simulink model "DS_distrIntp_4_0_realaxes"  (R2019b)
settings: Solver=FixedStepDiscrete  StartTime=0.0  StopTime=inf  FixedStep=Ts  RelTol=1e-3
StartFcn:
  | close all;
model workspace (MAT data in the model file):
  MvmtPerfEval_collectVal : Simulink.Parameter (value not decoded)
  MvmtPerfEval_sendOwnVal : Simulink.Parameter (value not decoded)
  PAR_center_c2 : Simulink.Parameter (value not decoded)
  PAR_numStepsAheadSmoothing : Simulink.Parameter (value not decoded)
  PAR_startPosReachedTol : Simulink.Parameter (value not decoded)
  PAR_workspace_c2 : Simulink.Parameter (value not decoded)
  PerfEval_numTicks_enable : Simulink.Parameter (value not decoded)
  Segmentregler_I_Gain : Simulink.Parameter (value not decoded)
  Segmentregler_P_Gain : Simulink.Parameter (value not decoded)
  Segmentregler_minVel_enable : Simulink.Parameter (value not decoded)
  Segmentregler_numTicks_enable : Simulink.Parameter (value not decoded)
  Ts : Simulink.Parameter (value not decoded)
  horizon : Simulink.Parameter (value not decoded)
  maxPos_x : Simulink.Parameter (value not decoded)
  maxPos_y : Simulink.Parameter (value not decoded)
  maxPos_z : Simulink.Parameter (value not decoded)
  maxVectorLengths : Simulink.Parameter (value not decoded)
  minAllowedVelSaturation : Simulink.Parameter (value not decoded)
  numAxes : Simulink.Parameter (value not decoded)
  window_length : Simulink.Parameter (value not decoded)
symbols that are objects in the model workspace (value not decoded): MvmtPerfEval_collectVal, MvmtPerfEval_sendOwnVal, numAxes, PAR_center_c2, PAR_numStepsAheadSmoothing, PAR_startPosReachedTol, PAR_workspace_c2, Ts
undefined symbols (not defined in the file or in its folder): DiscIntNeverNeededParam, setP_mat, VelOverride
libraries: vrlib x1, sldrtlib x1
(part 4 of 4)

== stateflow chart DS_distrIntp_4_0_realaxes/Achse X/Chart ==
  state Monitor_Inputs [parallel]
    settings: executionOrder=1
    state Wait
    state Update
      entry:
      send(newCommand);
    (default) -> Monitor_Inputs.Wait
    Monitor_Inputs.Wait -> Update : [hasChanged(ZielPos) ||...
        |  hasChanged(sollGeschw)]
    Update -> Monitor_Inputs.Wait
  state Exec_Commands [parallel]
    settings: executionOrder=2
    state Wait
      during:
      prevZielPos = ZielPos;
    state Send
      entry:
      if prevZielPos > ZielPos && sollGeschw ~= 0
      zP = ZielPos*1000-horizon;
      zP = max(zP,0);
      goToPos(PAR_isAxis,zP,sollGeschw);
      elseif prevZielPos < ZielPos && sollGeschw ~= 0
      zP = ZielPos*1000+horizon;
      goToPos(PAR_isAxis,zP,sollGeschw);
      elseif sollGeschw == 0
      zP = ZielPos *1000;
      goToPos(PAR_isAxis,zP,0.01);
      end
    state Send_after_Start
      % Hier geben wir bei noch icht initialisierter prevZielPos
      % KEINEN Horizont vor, da sonst falscher pos. Offset
      %im ersten Schritt
      entry:
      if prevZielPos > ZielPos && sollGeschw ~= 0
      goToPos(PAR_isAxis,zP,sollGeschw);
      elseif prevZielPos < ZielPos && sollGeschw ~= 0
      goToPos(PAR_isAxis,zP,sollGeschw);
      elseif sollGeschw == 0
      goToPos(PAR_isAxis,zP,0.01);
      end
      startFlag = 0;
    (default) -> Exec_Commands.Wait
    Exec_Commands.Wait -> Send [order 1] : newCommand[startFlag == 0]
    Send -> Exec_Commands.Wait
    Exec_Commands.Wait -> Send_after_Start [order 2] : newCommand
    Send_after_Start -> Exec_Commands.Wait
  state ReadPos [parallel]
    during:
    on every(5,tick): [Pos,TimeStamp] = getPos(PAR_isAxis);
    settings: executionOrder=3
  data: axis function_input; tPos function_input; tVel function_input; pos function_output; axis function_input; timeStamp function_output; ZielPos input; PAR_isAxis input; sollGeschw input; Pos output =0; TimeStamp output =0; prevZielPos local =0; zP local =0; horizon parameter; startFlag local =1
  events: newCommand local FUNCTION_CALL_EVENT
  function goToPos(axis,tPos,tVel):
    | function goToPos(axis,tPos,tVel)
    | 
    | coder.extrinsic('V_2_x_goToPos');
    | V_2_x_goToPos(axis,tPos,tVel);
    | 
    | 
    | end
  function [pos,timeStamp] = getPos(axis):
    | function [pos,timeStamp] = getPos(axis)
    | pos = 0;
    | timeStamp = 0;
    | 
    | coder.extrinsic('V_2_x_getPos');
    | %[pos] = V_2_x_getPos(axis);
    | [pos,timeStamp] = V_2_x_getPos(axis);
    | 
    | end

== stateflow chart DS_distrIntp_4_0_realaxes/Achse Y/Chart ==
  state Monitor_Inputs [parallel]
    settings: executionOrder=1
    state Wait
    state Update
      entry:
      send(newCommand);
    (default) -> Monitor_Inputs.Wait
    Monitor_Inputs.Wait -> Update : [hasChanged(ZielPos) ||...
        |  hasChanged(sollGeschw)]
    Update -> Monitor_Inputs.Wait
  state Exec_Commands [parallel]
    settings: executionOrder=2
    state Wait
      during:
      prevZielPos = ZielPos;
    state Send
      entry:
      if prevZielPos > ZielPos && sollGeschw ~= 0
      zP = ZielPos*1000-horizon;
      zP = max(zP,0);
      goToPos(PAR_isAxis,zP,sollGeschw);
      elseif prevZielPos < ZielPos && sollGeschw ~= 0
      zP = ZielPos*1000+horizon;
      goToPos(PAR_isAxis,zP,sollGeschw);
      elseif sollGeschw == 0
      zP = ZielPos *1000;
      goToPos(PAR_isAxis,zP,0.01);
      end
    state Send_after_Start
      % Hier geben wir bei noch icht initialisierter prevZielPos
      % KEINEN Horizont vor, da sonst falscher pos. Offset
      %im ersten Schritt
      entry:
      if prevZielPos > ZielPos && sollGeschw ~= 0
      goToPos(PAR_isAxis,zP,sollGeschw);
      elseif prevZielPos < ZielPos && sollGeschw ~= 0
      goToPos(PAR_isAxis,zP,sollGeschw);
      elseif sollGeschw == 0
      goToPos(PAR_isAxis,zP,0.01);
      end
      startFlag = 0;
    (default) -> Exec_Commands.Wait
    Exec_Commands.Wait -> Send [order 1] : newCommand[startFlag == 0]
    Send -> Exec_Commands.Wait
    Exec_Commands.Wait -> Send_after_Start [order 2] : newCommand
    Send_after_Start -> Exec_Commands.Wait
  state ReadPos [parallel]
    during:
    on every(5,tick): [Pos,TimeStamp] = getPos(PAR_isAxis);
    settings: executionOrder=3
  data: axis function_input; tPos function_input; tVel function_input; pos function_output; axis function_input; timeStamp function_output; ZielPos input; PAR_isAxis input; sollGeschw input; Pos output =0; TimeStamp output =0; prevZielPos local =0; zP local =0; horizon parameter; startFlag local =1
  events: newCommand local FUNCTION_CALL_EVENT
  function goToPos(axis,tPos,tVel):
    | function goToPos(axis,tPos,tVel)
    | 
    | coder.extrinsic('V_2_x_goToPos');
    | V_2_x_goToPos(axis,tPos,tVel);
    | 
    | 
    | end
  function [pos,timeStamp] = getPos(axis):
    | function [pos,timeStamp] = getPos(axis)
    | pos = 0;
    | timeStamp = 0;
    | 
    | coder.extrinsic('V_2_x_getPos');
    | %[pos] = V_2_x_getPos(axis);
    | [pos,timeStamp] = V_2_x_getPos(axis);
    | 
    | end

== stateflow chart DS_distrIntp_4_0_realaxes/Achse X/Achsgeschwindigkeit ==
  state new_measurement
    entry:
    if(oldTimeStamp) ~= 0
    delta_s = abs(Pos - oldPos);
    delta_t = TimeStamp - oldTimeStamp;
    velocity = delta_s / (delta_t / 1000);
    if sollGeschw ~= 0
    velocity_norm = velocity / (maxVelocity*0.8);
    else
    velocity_norm = 0;
    end
    end
  state Wait_for_new_measurement
    entry:
    oldPos = Pos;
    oldTimeStamp = TimeStamp;
  (default) -> Wait_for_new_measurement
  Wait_for_new_measurement -> new_measurement : [hasChanged(Pos) &&...
      |  hasChanged(TimeStamp)]
  new_measurement -> Wait_for_new_measurement
  data: Pos input; TimeStamp input; velocity output; delta_s local; delta_t local; oldPos local; oldTimeStamp local; velocity_norm output =0; maxVelocity input; sollGeschw input

== stateflow chart DS_distrIntp_4_0_realaxes/Achse Z/Achsgeschwindigkeit ==
  state new_measurement
    entry:
    if(oldTimeStamp) ~= 0
    delta_s = abs(Pos - oldPos);
    delta_t = TimeStamp - oldTimeStamp;
    velocity = delta_s / (delta_t / 1000);
    if sollGeschw ~= 0
    velocity_norm = velocity / (maxVelocity*0.8);
    else
    velocity_norm = 0;
    end
    end
  state Wait_for_new_measurement
    entry:
    oldPos = Pos;
    oldTimeStamp = TimeStamp;
  (default) -> Wait_for_new_measurement
  Wait_for_new_measurement -> new_measurement : [hasChanged(Pos) &&...
      |  hasChanged(TimeStamp)]
  new_measurement -> Wait_for_new_measurement
  data: Pos input; TimeStamp input; velocity output; delta_s local; delta_t local; oldPos local; oldTimeStamp local; velocity_norm output =0; maxVelocity input; sollGeschw input

== stateflow chart DS_distrIntp_4_0_realaxes/Achse Z/Chart ==
  state Monitor_Inputs [parallel]
    settings: executionOrder=1
    state Wait
    state Update
      entry:
      send(newCommand);
    (default) -> Monitor_Inputs.Wait
    Monitor_Inputs.Wait -> Update : [hasChanged(ZielPos) ||...
        |  hasChanged(sollGeschw)]
    Update -> Monitor_Inputs.Wait
  state Exec_Commands [parallel]
    settings: executionOrder=2
    note: Condition ggf. wieder einfügen startFlag == 0
    state Wait
      during:
      prevZielPos = ZielPos;
    state Send
      entry:
      if prevZielPos > ZielPos && sollGeschw ~= 0
      zP = ZielPos*1000-horizon;
      zP = max(zP,0);
      goToPos(PAR_isAxis,zP,sollGeschw);
      elseif prevZielPos < ZielPos && sollGeschw ~= 0
      zP = ZielPos*1000+horizon;
      goToPos(PAR_isAxis,zP,sollGeschw);
      elseif sollGeschw == 0
      zP = ZielPos *1000;
      goToPos(PAR_isAxis,zP,0.01);
      end
    state Send_after_Start [commented out]
      % Hier geben wir bei noch icht initialisierter prevZielPos
      % KEINEN Horizont vor, da sonst falscher pos. Offset
      %im ersten Schritt
      entry:
      if prevZielPos > ZielPos && sollGeschw ~= 0
      goToPos(PAR_isAxis,zP,sollGeschw);
      elseif prevZielPos < ZielPos && sollGeschw ~= 0
      goToPos(PAR_isAxis,zP,sollGeschw);
      elseif sollGeschw == 0
      goToPos(PAR_isAxis,zP,0.01);
      end
      startFlag = 0;
    (default) -> Exec_Commands.Wait
    Exec_Commands.Wait -> Send : newCommand
    Send -> Exec_Commands.Wait
    Exec_Commands.Wait -> Send_after_Start [commented out] : newCommand
    Send_after_Start -> Exec_Commands.Wait [commented out]
  state ReadPos [parallel]
    during:
    on every(5,tick): [Pos,TimeStamp] = getPos(PAR_isAxis);
    settings: executionOrder=3
  data: axis function_input; tPos function_input; tVel function_input; pos function_output; axis function_input; timeStamp function_output; ZielPos input; PAR_isAxis input; sollGeschw input; Pos output =0; TimeStamp output =0; prevZielPos local =0; zP local =0; horizon parameter; startFlag local =1
  events: newCommand local FUNCTION_CALL_EVENT
  function goToPos(axis,tPos,tVel):
    | function goToPos(axis,tPos,tVel)
    | 
    | coder.extrinsic('V_2_x_goToPos');
    | V_2_x_goToPos(axis,tPos,tVel);
    | 
    | 
    | end
  function [pos,timeStamp] = getPos(axis):
    | function [pos,timeStamp] = getPos(axis)
    | pos = 0;
    | timeStamp = 0;
    | 
    | coder.extrinsic('V_2_x_getPos');
    | %[pos] = V_2_x_getPos(axis);
    | [pos,timeStamp] = V_2_x_getPos(axis);
    | 
    | end

== stateflow chart DS_distrIntp_4_0_realaxes/Velocity GUI/Chart ==
  state Default
    during:
    %vel_x = GET_istGeschw(1);
    %vel_y = GET_istGeschw(2);
    %vel_z = GET_istGeschw(3);
    %vel_ges = sqrt(vel_x^2 + vel_y^2 + vel_z^2);
    vel_x_OR = VelOverride(1)*100;
    vel_y_OR = VelOverride(2)*100;
    vel_z_OR = VelOverride(3)*100;
    vel_c2_OR = VelOverride(4)*100;
    vel_ges = vecnorm(GET_normGeschw)*100;
    vel_ges_OR = vecnorm(VelOverride*100);
    vel_x_norm = min(GET_normGeschw(1)*100,vel_x_OR);
    vel_y_norm = min(GET_normGeschw(2)*100,vel_y_OR);
    vel_z_norm = min(GET_normGeschw(3)*100,vel_z_OR);
    vel_c2_norm = min(GET_normGeschw(4)*100,vel_c2_OR);
  (default) -> Default
  data: VelOverride data_store_memory; GET_istGeschw data_store_memory; GET_normGeschw data_store_memory; vel_ges output; vel_ges_OR output; vel_x_norm output; vel_y_norm output; vel_z_norm output; vel_x_OR output; vel_y_OR output; vel_z_OR output; vel_c2_OR output; vel_c2_norm output

== stateflow chart DS_distrIntp_4_0_realaxes/PosTracer ==
  state Wait_for_Init
  state Create_Plot
    entry:
    startPos = PS_createTracePlot(numAxes,PAR_workspace_c2./1000,PAR_center_c2./1000);
  state Fetch_Positions
    entry:
    for ii=1:size(GET_istPos,1)
    switch ii
    case 1
    pos_x = GET_istPos(ii);
    case 2
    pos_y = GET_istPos(ii);
    case 3
    pos_z = GET_istPos(ii);
    case 4
    pos_c2 = GET_istPos(ii);
    c2_RUN = 0 ~= GET_normGeschw(ii);
    case 5
    pos_x2 = GET_istPos(ii);
    end
    end
  state Update_Plot
    entry:
    if numAxes == 2
    PS_updateTracePlot(numAxes,pos_x,pos_y,0,0,0,FLAG_axesRunning,...
    PAR_workspace_c2,PAR_center_c2, c2_RUN);
    elseif numAxes == 3
    PS_updateTracePlot(numAxes,pos_x,pos_y,...
    pos_z,0,0,FLAG_axesRunning,PAR_workspace_c2,PAR_center_c2, c2_RUN);
    elseif numAxes == 4
    PS_updateTracePlot(numAxes,pos_x,pos_y,...
    pos_z,pos_c2,0,FLAG_axesRunning,PAR_workspace_c2,...
    PAR_center_c2, c2_RUN);
    elseif numAxes == 5
    PS_updateTracePlot(numAxes,pos_x,pos_y,...
    pos_z,pos_c2,pos_x2,FLAG_axesRunning,...
    PAR_workspace_c2,PAR_center_c2, c2_RUN);
    end
  state Update_Plot1 [commented out]
    entry:
    if numAxes == 2
    PS_updateTracePlot(numAxes,pos_x+startPos(1,1),pos_y+startPos(1,2),0,0,0,false,...
    PAR_workspace_c2./1000,PAR_center_c2./1000);
    elseif numAxes == 3
    PS_updateTracePlot(numAxes,pos_x+startPos(1,1),pos_y+startPos(1,2),...
    pos_z+startPos(1,3),0,0,true,PAR_workspace_c2./1000,PAR_center_c2./1000);
    elseif numAxes == 4
    PS_updateTracePlot(numAxes,pos_x+startPos(1,1),pos_y+startPos(1,2),...
    pos_z+startPos(1,3),pos_c2+startPos(1,4),0,true,PAR_workspace_c2./1000,...
    PAR_center_c2./1000);
    elseif numAxes == 5
    PS_updateTracePlot(numAxes,pos_x+startPos(1,1),pos_y+startPos(1,2),...
    pos_z+startPos(1,3),pos_c2+startPos(1,4),pos_x2+startPos(1,5),true,...
    PAR_workspace_c2./1000,PAR_center_c2./1000);
    end
  (default) -> Wait_for_Init
  Wait_for_Init -> Create_Plot : after(0.1,'sec')
  Create_Plot -> Fetch_Positions
  Fetch_Positions -> Update_Plot
  Update_Plot -> Fetch_Positions : after(15,tick)
  data: numAx function_input; sPos function_output; c2Workspace function_input; c2Center function_input; numAx function_input; pos1 function_input; pos2 function_input; pos3 function_input; pos4 function_input; pos5 function_input; drawLine function_input; c2Workspace function_input; c2Center function_input; c2_isRunning function_input; numAxes parameter; pos_x local =0; pos_y local =0; GET_istPos data_store_memory; pos_z local =0; startPos local size=[1 numAxes] =zeros(1,numAxes); ii local; bootstrapping_done local; pos_c2 local; pos_x2 local; PAR_center_c2 parameter; PAR_workspace_c2 parameter; GET_normGeschw data_store_memory; c2_RUN local; FLAG_axesRunning data_store_memory
  function sPos  = PS_createTracePlot(numAx,c2Workspace,c2Center):
    | function sPos  = PS_createTracePlot(numAx,c2Workspace,c2Center)
    | 
    | coder.extrinsic('evalin');
    | coder.extrinsic('setappdata');
    | 
    | setP = evalin('base','setP_mat');
    | 
    | sPos = zeros(1,numAx);
    | 
    | % x2Center = [450,75,1]; %x,y,z
    | % x2Workspace = [300,5,2]; %x-wide,y-wide,z-wide
    | 
    | % if(numAx == 5)
    | %     fig = figure;
    | %     ax = axes;
    | %         
    | %     [~,dim2,~] = size(setP);
    | %     plot3(ax,setP(1,1:dim2),setP(2,1:dim2),setP(3,1:dim2));
    | %     hold on
    | %     s = linspace(0,2*pi,50);
    | %     cX = [c2Center(1) (cos(s).*(c2Workspace(4)+c2Workspace(5))/2+c2Center(1))];
    | % 	cY = [c2Center(2) (-sin(s).*(c2Workspace(4)+c2Workspace(5))/2+c2Center(2))];
    | %     cZ = ones(1,length(cX)).*c2Center(3);
    | %     plot3(cX,cY,cZ);
    | %     hold on
    | %     x2X = linspace(x2Center(1)-x2Workspace(1)/2,x2Center(1)+x2Workspace(1)/2);
    | %     x2Y = ones(1,length(x2X)).*x2Center(2);
    | %     x2Z = ones(1,length(x2X)).*x2Center(3);
    | %     plot3(x2X,x2Y,x2Z); 
    | %     hold off
    | %     
    | %     
    | %     set(fig,'Tag','TraceFig');
    | %     set(ax,'Tag','TraceAxes');
    | %     set(ax,'NextPlot','add');
    | %     
    | %     sPos(1,1) = setP(1,1);
    | %     sPos(1,2) = setP(2,1);
    | %     sPos(1,3) = setP(3,1);
    | %     sPos(1,4) = 0;
    | %     sPos(1,5) = x2Center(1)-x2Workspace(1)/2;
    | %     
    | %     traceLine = plot3(ax,[setP(1,1) setP(1,1)],[setP(2,1) setP(2,1)],[setP(3,1) setP(3,1)],'Color',[0 0 1],'LineWidth',1);
    | %     setappdata(ax,'traceLine',traceLine);
    | 
    | if(numAx == 4)
    |     fig = figure;
    |     ax = axes;
    | 
    |         
    |     % Darstellung der Solltrajektorie
    |     [~,dim2,~] = size(setP);
    |     plot3(ax,setP(1,1:dim2),setP(2,1:dim2),setP(3,1:dim2),'k');
    | %     hold on
    |     set(ax,'NextPlot','add');  
    |     
    |     % Darstellung des RT
    |     s = linspace(0,2*pi,50);
    |     radius = (c2Workspace(4)+c2Workspace(5))/2;
    |     cX = [c2Center(1) (cos(s).*radius+c2Center(1))] .* 1000;
    | 	cY = [c2Center(2) (-sin(s).*radius+c2Center(2))] .* 1000;
    |     cZ1 = ones(1,length(cX)).*(c2Center(3)+c2Workspace(3)/2) .* 1000;
    |     plotKreis1 = plot3(ax,cX(2:end),cY(2:end),cZ1(2:end),'g', 'LineWidth', 5); 
    | %     hold off
    | %     cZ2 = ones(1,length(cX)).*(c2Center(3)-c2Workspace(3)/2) .* 1000;
    | %     plotKreis2 = plot3(ax,cX,cY,cZ2);
    |     
    |     set(fig,'Name','Verteilte Interpolation - DEVEKOS');
    |     set(fig, 'Position',  [0, 0, 1450, 1000]) % 1920 x 1080 px sind verfügbar
    |     set(fig,'MenuBar','none');
    |     set(fig,'ToolBar','none');
    |     set(ax, 'ZLim', [-0.01 0.08]) ;
    |     set(fig,'Tag','TraceFig');
    |     set(ax,'Tag','TraceAxes');
    |     set(ax,'ZDir','reverse');
    |     set(ax,'YDir','reverse');
    | 
    | 
    |     
    |     sPos(1,1) = setP(1,1);
    |     sPos(1,2) = setP(2,1);
    |     sPos(1,3) = setP(3,1);
    |     sPos(1,4) = 0;
    |     
    |     traceLine = plot3(ax,[setP(1,1) setP(1,1)],[setP(2,1) setP(2,1)],[setP(3,1) setP(3,1)],'Color',[0 0 1],'LineWidth',1);
    |     setappdata(ax,'traceLine',traceLine);
    | 
    | elseif(numAx == 3)
    |     fig = figure;
    |     ax = axes;
    |         
    |     [~,dim2,~] = size(setP);
    |     plot3(ax,setP(1,1:dim2),setP(2,1:dim2),setP(3,1:dim2));
    |     
    |     set(fig,'Tag','TraceFig');
    |     set(ax,'Tag','TraceAxes');
    |     set(ax,'NextPlot','add');
    |     
    |     sPos(1,1) = setP(1,1);
    |     sPos(1,2) = setP(2,1);
    |     sPos(1,3) = setP(3,1);
    |     
    |     traceLine = plot3(ax,[setP(1,1) setP(1,1)],[setP(2,1) setP(2,1)],[setP(3,1) setP(3,1)],'Color',[0 0 1],'LineWidth',1);
    |     setappdata(ax,'traceLine',traceLine);
    |     
    | elseif(numAx == 2)
    |     
    |     fig = figure;
    |     ax = axes;
    |         
    |     [~,dim2] = size(setP);
    |     plot(ax,setP(1,1:dim2),setP(2,1:dim2));
    |     
    |     set(fig,'Tag','TraceFig');
    |     set(ax,'Tag','TraceAxes');
    |     set(ax,'NextPlot','add');
    |     
    |     sPos(1,1) = setP(1,1);
    |     sPos(1,2) = setP(2,1);
    |     
    |     traceLine = plot(ax,[setP(1,1) setP(1,1)],[setP(2,1) setP(2,1)],'Color',[0 0 1],'LineWidth',1);
    |     setappdata(ax,'traceLine',traceLine);
    |     
    | end
    | 
    | 
    | end
  function PS_updateTracePlot(numAx,pos1,pos2,pos3,pos4,pos5,drawLine,c2Workspace,c2Center, c2_isRunning):
    | function PS_updateTracePlot(numAx,pos1,pos2,pos3,pos4,pos5,drawLine,c2Workspace,c2Center, c2_isRunning)
    | 
    | cRadius = (c2Workspace(4)+c2Workspace(5))/2;
    | markersize=75;
    | % x2Center = [450,75,1]; %x,y,z
    | % x2Workspace = [300,5,2]; %x-wide,y-wide,z-wide
    | 
    | coder.extrinsic('delete');
    | coder.extrinsic('scatter');
    | coder.extrinsic('scatter3');
    | coder.extrinsic('getappdata');
    | coder.extrinsic('setappdata');
    | 
    | ax = findobj('Tag','TraceAxes');
    | 
    | 
    | if(numAx >= 3)
    |     
    |     punkt = getappdata(ax,'tracePunkt');
    |     if isempty(punkt)
    |         punkt = scatter3(ax,pos1,pos2,pos3,markersize,'MarkerEdgeColor','r','LineWidth',2.5);
    |         setappdata(ax,'tracePunkt',punkt);
    |     else
    |         set(punkt,'XData',pos1);
    |         set(punkt,'YData',pos2);
    |         set(punkt,'ZData',pos3);
    |         if c2_isRunning
    |             set(punkt,'MarkerEdgeColor', 'g');
    |         else
    |             set(punkt,'MarkerEdgeColor', 'r');
    |         end
    |             
    |     end
    |     
    |     
    |     colvec=['m','r','g','b','y','k'];
    |     if (numAx >= 4)
    |         for i=1:6
    |             formatSpec = 'tracePunktC%d';
    |             punktC = getappdata(ax,sprintf(formatSpec,cast(i,'int8')));
    |             xKoord = c2Center(1) - cos((pos4+i*60-60)/180*pi)*cRadius;
    |             yKoord = -(c2Center(2) + sin((pos4+i*60-60)/180*pi)*cRadius)+2*c2Center(2);
    |             if isempty(punktC)
    |                 punktC = scatter3(ax,xKoord,yKoord,(c2Center(3)+c2Workspace(3)/2), markersize, 'MarkerEdgeColor','k','LineWidth',2.5);
    |                 setappdata(ax,sprintf(formatSpec,cast(i,'int8')),punktC);
    |             else
    |                 set(punktC,'XData',xKoord);
    |                 set(punktC,'YData',yKoord);
    |             end
    |             % SynchLine zeichnen
    |                 if drawLine && c2_isRunning
    |                     if  i == 5
    |                        synch = getappdata(ax,'synchLine');
    |                         if  isempty(synch)
    |                             synch = plot3(ax, [pos1, xKoord], [pos2, yKoord], [pos3, (c2Center(3)+c2Workspace(3)/2)],':g', 'LineWidth',2.5);
    |                             setappdata(ax,'synchLine',synch);
    |                         else
    |                             set(synch,'XData',[pos1, xKoord]);
    |                             set(synch,'YData',[pos2, yKoord]);
    |                             set(synch,'ZData',[pos3, (c2Center(3)+c2Workspace(3)/2)]);
    |                         end
    |                     end
    |                 else
    |                     synch = getappdata(ax,'synchLine');
    |         
    |                     set(synch,'XData',[]);
    |                     set(synch,'YData',[]);
    |                     set(synch,'ZData',[]);
    |                 end  
    | 
    |             
    |         end
    |         
    | %         if (numAx >= 5)
    | %             punktX2 = getappdata(ax,'tracePunktX2');
    | %             if isempty(punktX2)
    | %                 punktX2 = scatter3(ax,pos5,75,0,'MarkerEdgeColor','g','LineWidth',1.5);
    | %                 setappdata(ax,'tracePunktX2',punktX2);
    | %             else
    | %                 set(punktX2,'XData',pos5);
    | %             end
    | %         end
    |     end
    |     
    |     if drawLine
    |         
    |         traceLine = getappdata(ax,'traceLine');
    |         XData = get(traceLine,'XData');
    |         YData = get(traceLine,'YData');
    |         ZData = get(traceLine,'ZData');
    |         
    |         set(traceLine,'LineWidth',5);
    |         set(traceLine,'XData',[XData pos1]);
    |         set(traceLine,'YData',[YData pos2]);
    |         set(traceLine,'ZData',[ZData pos3]);
    |         
    |     else
    |         
    |         traceLine = getappdata(ax,'traceLine');
    |         
    |         set(traceLine,'XData',[]);
    |         set(traceLine,'YData',[]);
    |         set(traceLine,'ZData',[]);
    |         
    |     end
    |     
    | elseif(numAx == 2)
    |     
    |     punkt = scatter(ax,pos1,pos2,'MarkerEdgeColor','r','LineWidth',2);
    |     setappdata(ax,'tracePunkt',punkt);
    |     
    |     if drawLine
    |         
    |         traceLine = getappdata(ax,'traceLine');
    |         XData = get(traceLine,'XData');
    |         YData = get(traceLine,'YData');
    |         
    |         set(traceLine,'XData',[XData pos1]);
    |         set(traceLine,'YData',[YData pos2]);
    |         
    |     end   
    | end
    | end

== stateflow chart DS_distrIntp_4_0_realaxes/Joystick Ctrl/Chart ==
  state Idle
  state Start_interpolation
    entry:
    FLAG_startButton = true;
  state Stop_interpolation
    entry:
    FLAG_stopButton = true;
  note: Knopf
      | Zuordnung
      |
      | B(1)
      | Knopf A
      |
      | B(2)
      | Knopf B
      |
      | B(3)
      | Knopf X
      |
      | B(4)
      | Knopf Y
      |
      | B(5)
      | Knopf LB
      |
      | B(6)
      | Knopf RB
      |
      | B(7)
      | Knopf Reset
      |
      | B(8)
      | Knopf Start
      |
      | B(9)
      | Druckpunkt linker Stick
  note: Achse
      | Zuordnung
      |
      | A(1)
      | linker Stick (horizontal)
      |
      | A(2)
      | linker Stick (vertikal)
      |
      | A(3)
      | Trigger
      |
      | A(4)
      | rechter Stick (horizontal)
      |
      | A(5)
      | rechter Stick (vertikal)
  state Override_anpassen
    during:
    orX(1) = B(3)*A(3);
    orY(1) = B(4)*A(3);
    orZ(1) = B(1)*A(3);
    orC2(1) = B(2)*A(3);
    exit:
    orX(1) = 0;
    orY(1) = 0;
    orZ(1) = 0;
    orC2(1) = 0;
  state Override_gesamt_Reset
    entry:
    orX(2) = 1;
    orY(2) = 1;
    orZ(2) = 1;
    orC2(2) = 1;
    exit:
    orX(2) = 0;
    orY(2) = 0;
    orZ(2) = 0;
    orC2(2) = 0;
  state Override_Achse_Reset
    state axX
      entry:
      FLAG_resetAxis(1) = 1;
      FLAG_stopButton = true;
    state axY
      entry:
      FLAG_resetAxis(2) = 1;
      FLAG_stopButton = true;
    state axZ
      entry:
      FLAG_resetAxis(3) = 1;
      FLAG_stopButton = true;
    (junction 30) -> axZ [order 3] : [B(1)]
    (junction 30) -> axX [order 1] : [B(3)]
    (junction 30) -> axY [order 2] : [B(4)]
  (default) -> Idle
  Idle -> Start_interpolation [order 4] : [B(8) == 1]
  Start_interpolation -> Idle : [B(8) == 0]
  Idle -> Stop_interpolation [order 5] : [B(7) == 1]
  Stop_interpolation -> Idle : [B(7) == 0]
  Idle -> Override_anpassen [order 3] : [(B(1) || B(3) || B(4)) || B(2) && B(5) ~=1 && B(6)~=1]
  Override_anpassen -> Idle : [B(1)==0 && B(3)==0 && B(4)==0 && B(2) == 0]
  Idle -> Override_gesamt_Reset [order 2] : [B(9)]
  Override_gesamt_Reset -> Idle
  Idle -> (junction 30) [order 1] : [B(5) && B(6)]
  Override_Achse_Reset -> Idle : [B(5) == 0 || B(6) == 0]
  data: A input; orX output size=[1 2] =[0 0]; B input; orY output size=[1 2] =[0 0]; orZ output size=[1,2] =[0 0]; FLAG_startButton data_store_memory; FLAG_stopButton data_store_memory; FLAG_resetAxis data_store_memory; orC2 output size=[1,2] =[0 0]

== stateflow chart DS_distrIntp_4_0_realaxes/Joystick Ctrl/Chart1 ==
  state Idle
    JoystickTT();
  note: Knopf
      | Zuordnung
      |
      | B(1)
      | Knopf A
      |
      | B(2)
      | Knopf B
      |
      | B(3)
      | Knopf X
      |
      | B(4)
      | Knopf Y
      |
      | B(5)
      | Knopf LB
      |
      | B(6)
      | Knopf RB
      |
      | B(7)
      | Knopf Reset
      |
      | B(8)
      | Knopf Start
  note: Achse
      | Zuordnung
      |
      | A(1)
      | linker Stick (horizontal)
      |
      | A(2)
      | linker Stick (vertikal)
      |
      | A(3)
      | Trigger
      |
      | A(4)
      | rechter Stick (horizontal)
      |
      | A(5)
      | rechter Stick (vertikal)
  (default) -> Idle
  data: A input; orX output size=[1 2] =[0 0]; B input; orY output size=[1 2] =[0 0]; orZ output size=[1,2] =[0 0]; FLAG_stopButton data_store_memory; FLAG_startButton data_store_memory
  function JoystickTT:
    | function JoystickTT
    | 
    | aVarTruthTableCondition_1 = false;
    | aVarTruthTableCondition_2 = false;
    | aVarTruthTableCondition_3 = false;
    | aVarTruthTableCondition_4 = false;
    | aVarTruthTableCondition_5 = false;
    | aVarTruthTableCondition_6 = false;
    | aVarTruthTableCondition_7 = false;
    | aVarTruthTableCondition_8 = false;
    | 
    | 
    | % Knopf X
    | % (x-Achse)
    | 
    | aVarTruthTableCondition_1 = logical(B(3));
    | 
    | % Knopf Y
    | % (y-Achse)
    | 
    | aVarTruthTableCondition_2 = logical(B(4));
    | 
    | % Knopf A
    | % (z-Achse)
    | 
    | aVarTruthTableCondition_3 = logical(B(1));
    | 
    | % Knopf B
    | 
    | aVarTruthTableCondition_4 = logical(B(2));
    | 
    | % Knopf LB
    | 
    | aVarTruthTableCondition_5 = logical(B(5));
    | 
    | % Knopf RB
    | 
    | aVarTruthTableCondition_6 = logical(B(6));
    | 
    | % Knopf RESET
    | 
    | aVarTruthTableCondition_7 = logical(B(7));
    | 
    | % Knopf START
    | 
    | aVarTruthTableCondition_8 = logical(B(8));
    | 
    | if (aVarTruthTableCondition_1 && ~aVarTruthTableCondition_4 && ~aVarTruthTableCondition_5 && ~aVarTruthTableCondition_6 && ~aVarTruthTableCondition_7 && ~aVarTruthTableCondition_8)
    |     a2();
    | elseif (aVarTruthTableCondition_2 && ~aVarTruthTableCondition_4 && ~aVarTruthTableCondition_5 && ~aVarTruthTableCondition_6 && ~aVarTruthTableCondition_7 && ~aVarTruthTableCondition_8)
    |     a2();
    | elseif (aVarTruthTableCondition_3 && ~aVarTruthTableCondition_4 && ~aVarTruthTableCondition_5 && ~aVarTruthTableCondition_6 && ~aVarTruthTableCondition_7 && ~aVarTruthTableCondition_8)
    |     a2();
    | elseif (~aVarTruthTableCondition_1 && ~aVarTruthTableCondition_2 && ~aVarTruthTableCondition_3 && aVarTruthTableCondition_4 && ~aVarTruthTableCondition_5 && ~aVarTruthTableCondition_6 && ~aVarTruthTableCondition_7 && ~aVarTruthTableCondition_8)
    |     a3();
    | elseif (aVarTruthTableCondition_1 && ~aVarTruthTableCondition_2 && ~aVarTruthTableCondition_3 && ~aVarTruthTableCondition_4 && aVarTruthTableCondition_5 && aVarTruthTableCondition_6 && ~aVarTruthTableCondition_7 && ~aVarTruthTableCondition_8)
    |     a4();
    | elseif (~aVarTruthTableCondition_1 && aVarTruthTableCondition_2 && ~aVarTruthTableCondition_3 && ~aVarTruthTableCondition_4 && aVarTruthTableCondition_5 && aVarTruthTableCondition_6 && ~aVarTruthTableCondition_7 && ~aVarTruthTableCondition_8)
    |     a5();
    | elseif (~aVarTruthTableCondition_1 && ~aVarTruthTableCondition_2 && aVarTruthTableCondition_3 && ~aVarTruthTableCondition_4 && aVarTruthTableCondition_5 && aVarTruthTableCondition_6 && ~aVarTruthTableCondition_7 && ~aVarTruthTableCondition_8)
    |     a6();
    | elseif (aVarTruthTableCondition_7)
    |     s();
    | elseif (aVarTruthTableCondition_8)
    |     go();
    | else % Default
    |     null();
    | end
    | 
    | function null()
    | 
    | % null
    | 
    | FLAG_startButton = false;
    | FLAG_stopButton = false;
    | orX = zeros(1,2);
    | orY = zeros(1,2);
    | orZ = zeros(1,2);
    | orX(2) = 0;
    | orY(2) = 0;
    | orZ(2) = 0;
    | 
    | function go()
    | 
    | % StartSimulation
    | 
    | FLAG_startButton = true;
    | 
    | function s()
    | 
    | % StopSimulation
    | 
    | FLAG_stopButton = true;
    | 
    | function a2()
    | 
    | % oR anpassen
    | 
    | orX(1) = B(3)*A(3);
    | orY(1) = B(4)*A(3);
    | orZ(1) = B(1)*A(3);
    | 
    | function a3()
    | 
    | % oR Reset für alle Achsen
    | 
    | orX(2) = 1;
    | orY(2) = 1;
    | orZ(2) = 1;
    | 
    | function a4()
    | 
    | % oR Reset für x-Achse
    | 
    | orX(2) = 1;
    | 
    | function a5()
    | 
    | % oR Reset für y-Achse
    | 
    | orY(2) = 1;
    | 
    | function a6()
    | 
    | % oR Reset für z-Achse
    | 
    | orZ(2) = 1;

== stateflow chart DS_distrIntp_4_0_realaxes/Achse C2/Chart ==
  state Monitor_Inputs [parallel]
    settings: executionOrder=1
    state Wait
    state Update
      entry:
      ff = 1;
      send(newCommand);
      exit:
      ff = 0;
    (default) -> Monitor_Inputs.Wait
    Monitor_Inputs.Wait -> Update : [hasChanged(ZielPos) ||...
        |  hasChanged(sollGeschw)]
    Update -> Monitor_Inputs.Wait
  state Exec_Commands [parallel]
    settings: executionOrder=2
    state Send
      entry:
      goToPos(ZielPos,sollGeschw);
    state Wait
      during:
      prevZielPos = ZielPos;
    (default) -> Exec_Commands.Wait
    Exec_Commands.Wait -> Send : newCommand
    Send -> Exec_Commands.Wait
  state ReadPos [parallel]
    during:
    on every(5,tick): Pos = getPos();
    settings: executionOrder=3
  data: pos function_input; vel function_input; pos function_output; ZielPos input; PAR_isAxis input; sollGeschw input; Pos output =0; prevZielPos local =0; ff local =0
  events: newCommand local FUNCTION_CALL_EVENT
  function goToPos(pos,vel):
    | function goToPos(pos,vel)
    | 
    | coder.extrinsic('PS_Hiwin_goToPos');
    | PS_Hiwin_goToPos(pos,vel);
    | 
    | 
    | end
  function pos  = getPos:
    | function pos  = getPos
    | pos = 0;
    | 
    | coder.extrinsic('PS_Hiwin_getPos');
    | pos = PS_Hiwin_getPos();
    | 
    | end

== stateflow chart DS_distrIntp_4_0_realaxes/Achse C2/Achsgeschwindigkeit ==
  state new_measurement
    entry:
    if(sollGeschw ~= 0)
    v = getVel();
    v_norm = 100*(v / (max_vel*0.8));
    else
    v_norm = 0;
    end
  state Wait_for_new_measurement
  (default) -> Wait_for_new_measurement
  Wait_for_new_measurement -> new_measurement : [hasChanged(Pos)]
  new_measurement -> Wait_for_new_measurement
  data: vel function_output; Pos input; v output; max_vel input; v_norm output; sollGeschw input
  function vel  = getVel:
    | function vel  = getVel
    | vel = 0;
    | 
    | coder.extrinsic('PS_Hiwin_getVel');
    | vel = PS_Hiwin_getVel();
    | 
    | end
